simulink model "winter_simulink_drawings"  (R2022a)
settings: Solver=FixedStepAuto  StartTime=0  StopTime=simulation.stop_time  FixedStep=simulation.time_step  RelTol=1e-3
values from neighbouring files (symbols this model uses):
  Gc = 1/(1 + s*tau_c)    [PMSM_TF.m]    (also in PMSM_TF_pid.m; generator_test.m; tuning_example.m)
  I_eq = rotor.I + generator.I/gearbox.ratio^2    [parameters.m]
  Lambda = generator.Lambda    [PMSM_TF.m]    (also in PMSM_TF_pid.m; generator_test.m; tuning_example.m)
  lambda_vector = linspace(lambda_range(1), lambda_range(2), lambda_item)    [parameters.m]
  n = gearbox.ratio    [generator_test.m]    (also in tuning_example.m)
  omega_rated = rated_values(2)    [parameters.m]
  p = generator.p    [PMSM_TF.m]    (also in PMSM_TF_pid.m; generator_test.m; tuning_example.m)
  pitch_range = deg2rad([-15 90])    [parameters.m]
  pitch_vector = linspace(pitch_range(1), pitch_range(2), pitch_item)    [parameters.m]
  rho = 1.225    [parameters.m]
  Riq = (Riq_pid.kp + Riq_pid.ki/s)    [PMSM_TF.m]    (also in PMSM_TF_pid.m = (Riq_pid.kp + Riq_pid.ki/s + Riq_pid.kd*s)*(1/(1 + s/(2*iq_o; generator_test.m = kiq_p + 1/s*kiq_i + s*kiq_d)
  wind_speed = run_generated_wind_series(wind.mean(i),          wind.turbulence(i), wind_speed, stop_time)    [main.m]    (also in rotor_test.m = 25)
  Yiq = (B+s*I)/(L*I*s^2+(R*I+L*B)*s+R*B+1.5*(p*Lambda)^2)    [PMSM_TF.m]    (also in PMSM_TF_pid.m; generator_test.m; tuning_example.m)
undefined symbols (not defined in the file or in its folder): blade, gearbox, generator, K_opt, lookup_cP, M_R, omega_r, rotor, wind
settings Model: Creator=Niccolò  LastModifiedBy=Niccolò

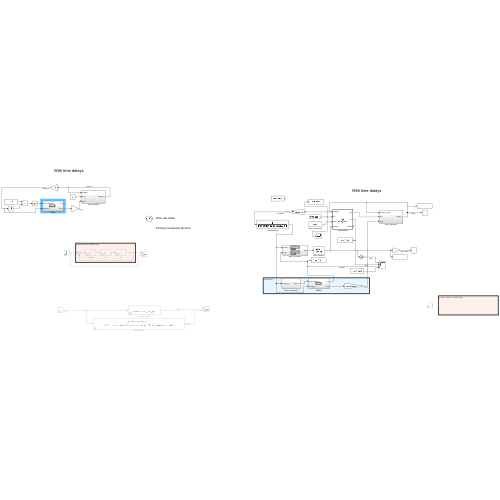
[thumbnail: Simulink's stored preview of the top-level diagram]
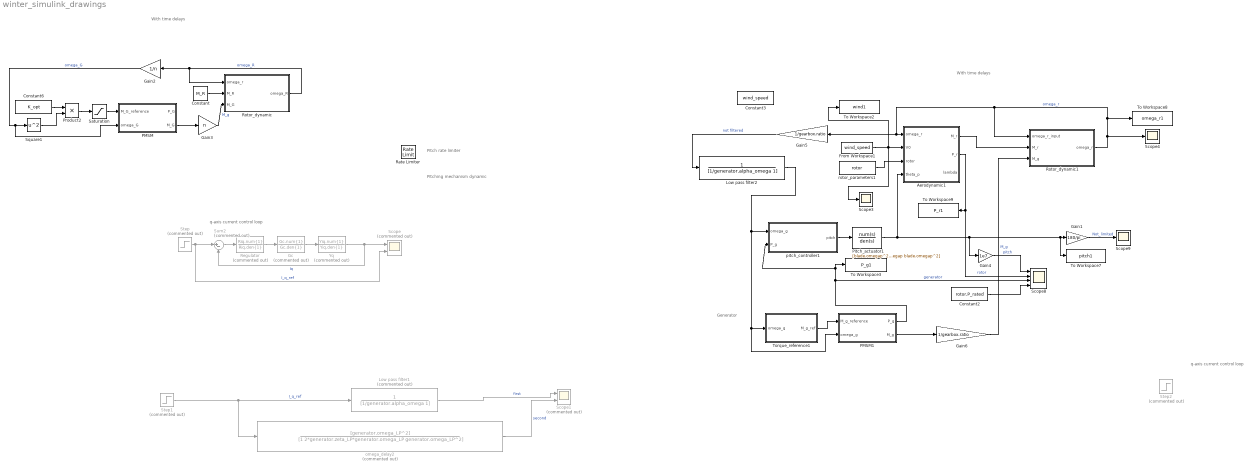
== system winter_simulink_drawings ==
  note: Pitching mechanism dynamic
  note: Pitch rate limiter
  note: With time delays
  note: q-axis current control loop
  note: q-axis current control loop
  note: Generator
  note: With time delays
  Aerodynamic1 : MATLAB Function  TreatAsAtomicUnit=on
  Constant : Constant  Value=M_R
  Constant2 : Constant  Value=rotor.P_rated
  Constant3 : Constant  Value=wind_speed
  Constant6 : Constant  Value=K_opt
  From Workspace1 : FromWorkspace  VariableName=wind_speed  SampleTime=1/wind.sample_f
  Gain1 : Gain  Gain=180/pi
  Gain2 : Gain  Gain=1/n
  Gain3 : Gain  Gain=n
  Gain4 : Gain  Gain=1e7
  Gain5 : Gain  Gain=1/gearbox.ratio
  Gain6 : Gain  Gain=1/gearbox.ratio
  Gc : TransferFcn  Commented=on  Numerator=Gc.num{1}  Denominator=Gc.den{1}
  Low pass filter1 : TransferFcn  Commented=on  Denominator=[1/generator.alpha_omega 1]
  Low pass filter2 : TransferFcn  Denominator=[1/generator.alpha_omega 1]
  PMSM : Subsystem
  PMSM1 : Subsystem
  Pitch_actuator1 : TransferFcn  Numerator=[blade.omegap^2]  Denominator=[1 2*blade.zetap*blade.omegap blade.omegap^2]
  Product2 : Product
  Rate Limiter : RateLimiter  RisingSlewLimit=blade.pitch_rate  FallingSlewLimit=-blade.pitch_rate  SampleTimeMode=inherited
  Regulator : TransferFcn  Commented=on  Numerator=Riq.num{1}  Denominator=Riq.den{1}
  Rotor_dynamic : Subsystem
  Rotor_dynamic1 : Subsystem
  Saturation : Saturate  UpperLimit=0  LowerLimit=0
  Scope : Scope  Commented=on  NumInputPorts=2
  Scope1 : Scope  Commented=on  NumInputPorts=2
  Scope3 : Scope
  Scope4 : Scope
  Scope8 : Scope  NumInputPorts=4
  Scope9 : Scope
  Square1 : Math  Operator=square
  Step : Step  Commented=on  SampleTime=0
  Step1 : Step  Commented=on  SampleTime=0
  Step2 : Step  Commented=on  SampleTime=0
  Sum2 : Sum  Commented=on  Inputs=|+-
  To Workspace2 : ToWorkspace  VariableName=wind1  SaveFormat=Timeseries  SampleTime=-1
  To Workspace3 : ToWorkspace  VariableName=P_g1  SaveFormat=Timeseries  SampleTime=-1
  To Workspace7 : ToWorkspace  VariableName=pitch1  SaveFormat=Timeseries  SampleTime=-1
  To Workspace8 : ToWorkspace  VariableName=omega_r1  SaveFormat=Timeseries  SampleTime=-1
  To Workspace9 : ToWorkspace  VariableName=P_r1  SaveFormat=Timeseries  SampleTime=-1
  Torque_reference1 : Subsystem
  Yq : TransferFcn  Commented=on  Numerator=Yiq.num{1}  Denominator=Yiq.den{1}
  omega_delay2 : TransferFcn  Commented=on  Numerator=[generator.omega_LP^2]  Denominator=[1 2*generator.zeta_LP*generator.omega_LP generator.omega_LP^2]
  pitch_controller1 : Subsystem
  rotor_parameters1 : Constant  Value=rotor  OutDataTypeStr=Bus: rotor_bus
  wires:
  Gain2/1 -> PMSM/2(omega_G), Square1/1  "omega_G"
  Rotor_dynamic/1(omega_R) -> Gain2/1, Rotor_dynamic/1(omega_r)  "omega_R"
  Saturation/1 -> PMSM/1(M_G_reference)
  PMSM/2(M_G) -> Gain3/1
  Gain3/1 -> Rotor_dynamic/3(M_G)  "M_g"
  Step/1 -> Scope/2, Sum2/1  "I_q_ref"
  Gc/1 -> Yq/1
  Regulator/1 -> Gc/1
  Yq/1 -> Scope/1, Sum2/2  "Iq"
  Sum2/1 -> Regulator/1
  Step1/1 -> omega_delay2/1, Low pass filter1/1  "I_q_ref"
  Low pass filter1/1 -> Scope1/1  "first"
  omega_delay2/1 -> Scope1/2  "second"
  Torque_reference1/1(M_g_ref) -> PMSM1/1(M_g_reference)
  Gain4/1 -> Scope8/1  "pitch"
  Gain1/1 -> Scope9/1  "Not_limited"
  Low pass filter2/1 -> PMSM1/2(omega_g), Torque_reference1/1(omega_g), pitch_controller1/1(omega_g)
  pitch_controller1/1(pitch) -> Pitch_actuator1/1
  Gain6/1 -> Rotor_dynamic1/3(M_g)  "M_g"
  Rotor_dynamic1/1(omega_r) -> Scope4/1, To Workspace8/1, Rotor_dynamic1/1(omega_r_input), Gain5/1, Aerodynamic1/1(omega_r)  "omega_r"
  rotor_parameters1/1 -> Aerodynamic1/3(rotor)
  Gain5/1 -> Low pass filter2/1  "not filtered"
  Aerodynamic1/1(M_r) -> Rotor_dynamic1/2(M_r)
  Aerodynamic1/2(P_r) -> Scope8/2, To Workspace9/1  "rotor"
  Pitch_actuator1/1 -> To Workspace7/1, Gain1/1, Gain4/1, Aerodynamic1/4(theta_p)
  PMSM1/2(M_g) -> Gain6/1
  From Workspace1/1 -> Scope3/1, To Workspace2/1, Aerodynamic1/2(V0)
  PMSM1/1(P_g) -> To Workspace3/1, pitch_controller1/2(P_g), Scope8/3  "generator"
  Constant2/1 -> Scope8/4
  Constant6/1 -> Product2/1
  Square1/1 -> Product2/2
  Product2/1 -> Saturation/1
  Constant/1 -> Rotor_dynamic/2(M_R)

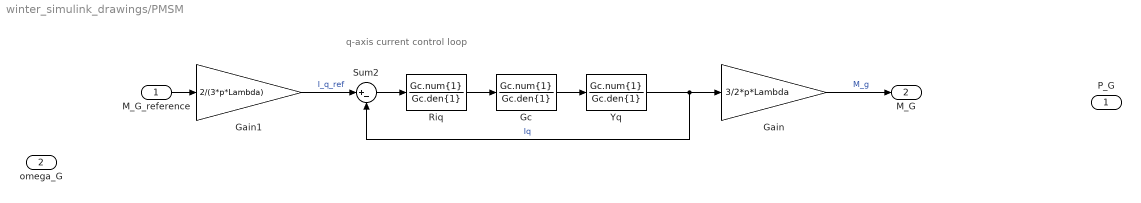
== system winter_simulink_drawings/PMSM ==
  note: q-axis current control loop
  M_G_reference : Inport
  omega_G : Inport  Port=2
  Gain : Gain  Gain=3/2*p*Lambda
  Gain1 : Gain  Gain=2/(3*p*Lambda)
  Gc : TransferFcn  Numerator=Gc.num{1}  Denominator=Gc.den{1}
  Riq : TransferFcn  Numerator=Gc.num{1}  Denominator=Gc.den{1}
  Sum2 : Sum  Inputs=|+-
  Yq : TransferFcn  Numerator=Gc.num{1}  Denominator=Gc.den{1}
  P_G : Outport
  M_G : Outport  Port=2
  wires:
  Gc/1 -> Yq/1
  M_G_reference/1 -> Gain1/1
  Gain/1 -> M_G/1  "M_g"
  Riq/1 -> Gc/1
  Sum2/1 -> Riq/1
  Yq/1 -> Gain/1, Sum2/2  "Iq"
  Gain1/1 -> Sum2/1  "I_q_ref"

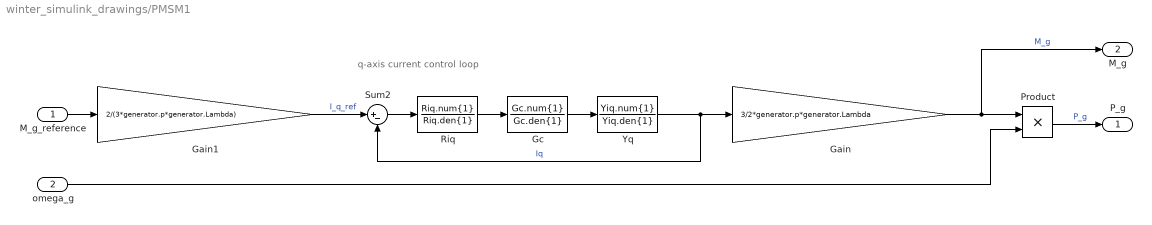
== system winter_simulink_drawings/PMSM1 ==
  note: q-axis current control loop
  M_g_reference : Inport
  omega_g : Inport  Port=2
  Gain : Gain  Gain=3/2*generator.p*generator.Lambda
  Gain1 : Gain  Gain=2/(3*generator.p*generator.Lambda)
  Gc : TransferFcn  Numerator=Gc.num{1}  Denominator=Gc.den{1}
  Product : Product
  Riq : TransferFcn  Numerator=Riq.num{1}  Denominator=Riq.den{1}
  Sum2 : Sum  Inputs=|+-
  Yq : TransferFcn  Numerator=Yiq.num{1}  Denominator=Yiq.den{1}
  P_g : Outport
  M_g : Outport  Port=2
  wires:
  Gc/1 -> Yq/1
  M_g_reference/1 -> Gain1/1
  Gain/1 -> M_g/1, Product/1  "M_g"
  Riq/1 -> Gc/1
  Sum2/1 -> Riq/1
  Yq/1 -> Gain/1, Sum2/2  "Iq"
  Product/1 -> P_g/1  "P_g"
  omega_g/1 -> Product/2
  Gain1/1 -> Sum2/1  "I_q_ref"

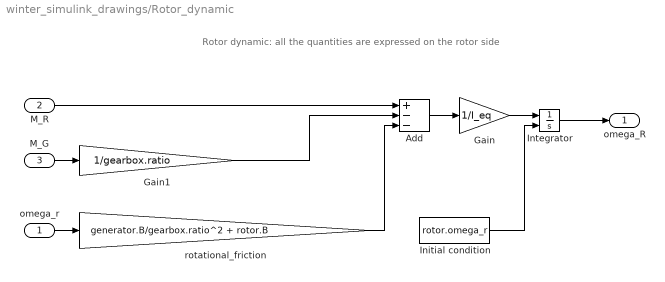
== system winter_simulink_drawings/Rotor_dynamic ==
  note: Rotor dynamic: all the quantities are expressed on the rotor side
  omega_r : Inport
  M_R : Inport  Port=2
  M_G : Inport  Port=3
  Add : Sum  Inputs=+--
  Gain : Gain  Gain=1/I_eq
  Gain1 : Gain  Gain=1/gearbox.ratio
  Initial condition : Constant  Value=rotor.omega_r
  Integrator : Integrator  InitialConditionSource=external  InitialCondition=omega_r
  rotational_friction : Gain  Gain=generator.B/gearbox.ratio^2 + rotor.B
  omega_R : Outport
  wires:
  Add/1 -> Gain/1
  Gain/1 -> Integrator/1
  M_R/1 -> Add/1
  Initial condition/1 -> Integrator/2
  omega_r/1 -> rotational_friction/1
  rotational_friction/1 -> Add/3
  M_G/1 -> Gain1/1
  Gain1/1 -> Add/2
  Integrator/1 -> omega_R/1

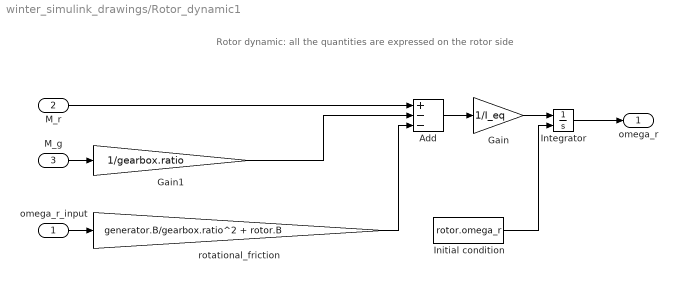
== system winter_simulink_drawings/Rotor_dynamic1 ==
  note: Rotor dynamic: all the quantities are expressed on the rotor side
  omega_r_input : Inport
  M_r : Inport  Port=2
  M_g : Inport  Port=3
  Add : Sum  Inputs=+--
  Gain : Gain  Gain=1/I_eq
  Gain1 : Gain  Gain=1/gearbox.ratio
  Initial condition : Constant  Value=rotor.omega_r
  Integrator : Integrator  InitialConditionSource=external  InitialCondition=omega_r
  rotational_friction : Gain  Gain=generator.B/gearbox.ratio^2 + rotor.B
  omega_r : Outport
  wires:
  Add/1 -> Gain/1
  Gain/1 -> Integrator/1
  M_r/1 -> Add/1
  Initial condition/1 -> Integrator/2
  omega_r_input/1 -> rotational_friction/1
  rotational_friction/1 -> Add/3
  M_g/1 -> Gain1/1
  Gain1/1 -> Add/2
  Integrator/1 -> omega_r/1

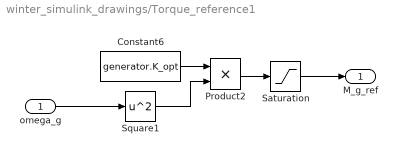
== system winter_simulink_drawings/Torque_reference1 ==
  omega_g : Inport
  Constant6 : Constant  Value=generator.K_opt
  Product2 : Product
  Saturation : Saturate  UpperLimit=rotor.P_rated*gearbox.ratio/omega_rated  LowerLimit=0
  Square1 : Math  Operator=square
  M_g_ref : Outport
  wires:
  Product2/1 -> Saturation/1
  omega_g/1 -> Square1/1
  Square1/1 -> Product2/2
  Constant6/1 -> Product2/1
  Saturation/1 -> M_g_ref/1

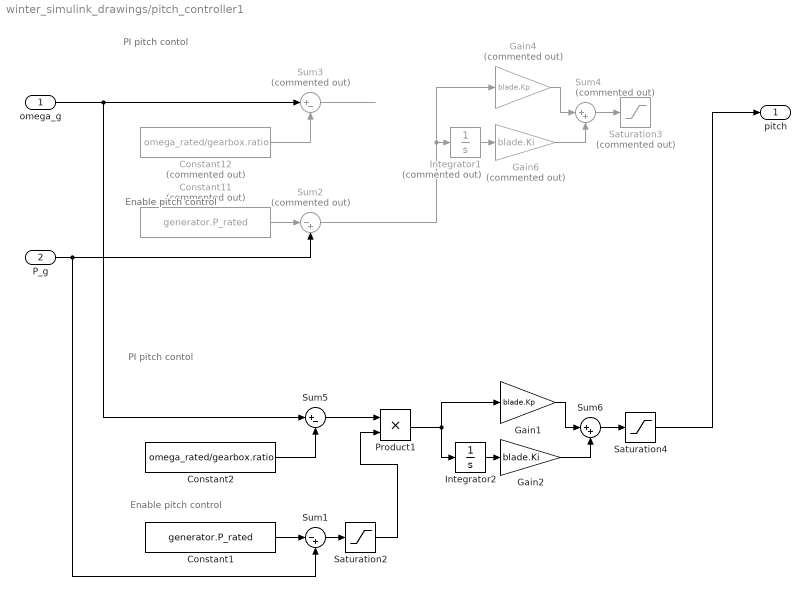
== system winter_simulink_drawings/pitch_controller1 ==
  note: PI pitch contol
  note: Enable pitch control
  note: Enable pitch control
  note: PI pitch contol
  omega_g : Inport
  P_g : Inport  Port=2
  Constant1 : Constant  Value=generator.P_rated
  Constant11 : Constant  Commented=on  Value=generator.P_rated
  Constant12 : Constant  Commented=on  Value=omega_rated/gearbox.ratio
  Constant2 : Constant  Value=omega_rated/gearbox.ratio
  Gain1 : Gain  Gain=blade.Kp
  Gain2 : Gain  Gain=blade.Ki
  Gain4 : Gain  Commented=on  Gain=blade.Kp
  Gain6 : Gain  Commented=on  Gain=blade.Ki
  Integrator1 : Integrator  Commented=on
  Integrator2 : Integrator
  Product1 : Product
  Saturation2 : Saturate  UpperLimit=1  LowerLimit=0
  Saturation3 : Saturate  Commented=on  UpperLimit=pitch_range(2)  LowerLimit=0
  Saturation4 : Saturate  UpperLimit=pitch_range(2)  LowerLimit=pitch_range(1)
  Sum1 : Sum  Inputs=|-+
  Sum2 : Sum  Commented=on  Inputs=|-+
  Sum3 : Sum  Commented=on  Inputs=|+-
  Sum4 : Sum  Commented=on  Inputs=|++
  Sum5 : Sum  Inputs=|+-
  Sum6 : Sum  Inputs=|++
  pitch : Outport
  wires:
  Constant11/1 -> Sum2/1
  Gain4/1 -> Sum4/1
  Sum2/1 -> Gain4/1, Integrator1/1
  Integrator1/1 -> Gain6/1
  Gain6/1 -> Sum4/2
  Constant12/1 -> Sum3/2
  Sum4/1 -> Saturation3/1
  Sum3/1 -> ?
  Saturation4/1 -> pitch/1
  omega_g/1 -> Sum5/1, Sum3/1
  Sum5/1 -> Product1/1
  Sum1/1 -> Saturation2/1
  P_g/1 -> Sum1/2, Sum2/2
  Sum6/1 -> Saturation4/1
  Gain1/1 -> Sum6/1
  Gain2/1 -> Sum6/2
  Integrator2/1 -> Gain2/1
  Constant2/1 -> Sum5/2
  Constant1/1 -> Sum1/1
  Product1/1 -> Integrator2/1, Gain1/1
  Saturation2/1 -> Product1/2

== matlab function winter_simulink_drawings/Aerodynamic1 ==
  data: omega_r input; V0 input; M_r output; P_r output; rho parameter; rotor input; theta_p input; lambda_vector parameter; pitch_vector parameter; lookup_cP parameter; lambda output
function [M_r, P_r, lambda] = Aerodynamic(omega_r, V0, rho, rotor, ...
  theta_p, lambda_vector, pitch_vector, lookup_cP) 

R = rotor.R;                  % rotor radius [m]

% retrive the cP from the look-up table
lambda = omega_r*R/V0;                                                
cP = interp2(lambda_vector, pitch_vector, lookup_cP, lambda, theta_p);

P_r = 0.5*rho*V0^3*pi*R^2*cP; % rotor power [W]
M_r = P_r/omega_r;            % rotor torque [Nm]
